simulink model "Timer_mdl"  (R2022b)
settings: Solver=FixedStepAuto  StartTime=0.0  StopTime=20  FixedStep=.01  RelTol=1e-3
settings Model: Creator=Sajjad  LastModifiedBy=Sajjad

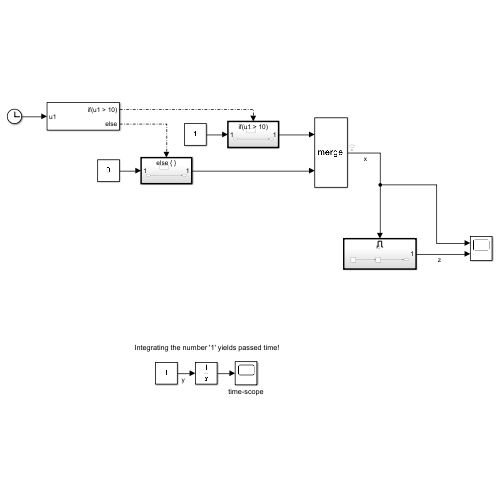
[thumbnail: Simulink's stored preview of the top-level diagram]
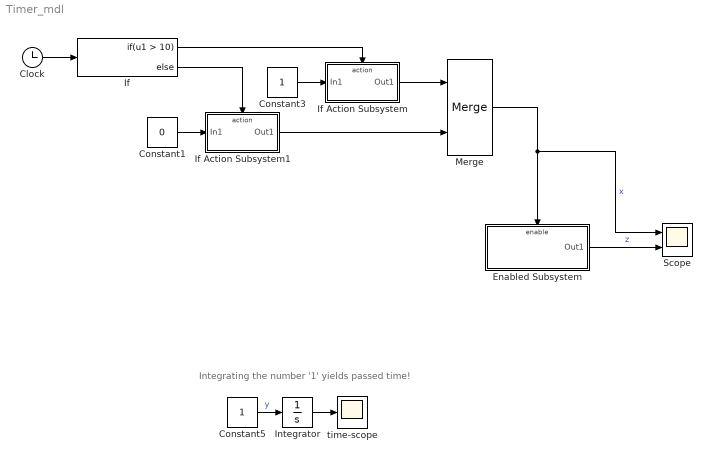
== system Timer_mdl ==
  note: Integrating the number '1' yields passed time!
  Clock : Clock
  Constant1 : Constant  Value=0
  Constant3 : Constant
  Constant5 : Constant
  Enabled Subsystem : Subsystem  TreatAsAtomicUnit=on
  If : If  IfExpression=u1 > 10
  If Action Subsystem : Subsystem  TreatAsAtomicUnit=on
  If Action Subsystem1 : Subsystem  TreatAsAtomicUnit=on
  Integrator : Integrator
  Merge : Merge
  Scope : Scope  NumInputPorts=2
  time-scope : Scope
  wires:
  Merge/1 -> Enabled Subsystem/Enable, Scope/1  "x"
  Clock/1 -> If/1
  If/1 -> If Action Subsystem/Action
  If/2 -> If Action Subsystem1/Action
  If Action Subsystem/1(Out1) -> Merge/1
  If Action Subsystem1/1(Out1) -> Merge/2
  Constant1/1 -> If Action Subsystem1/1(In1)
  Constant3/1 -> If Action Subsystem/1(In1)
  Constant5/1 -> Integrator/1  "y"
  Integrator/1 -> time-scope/1
  Enabled Subsystem/1(Out1) -> Scope/2  "z"

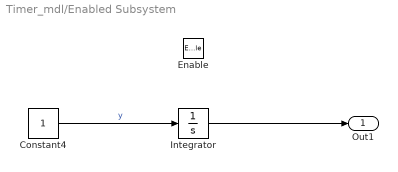
== system Timer_mdl/Enabled Subsystem ==
  Enable : EnablePort
  Constant4 : Constant
  Integrator : Integrator
  Out1 : Outport
  wires:
  Constant4/1 -> Integrator/1  "y"
  Integrator/1 -> Out1/1

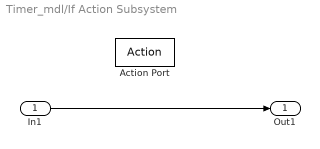
== system Timer_mdl/If Action Subsystem ==
  In1 : Inport
  Action Port : ActionPort  ActionPortLabel=if(u1 > 10)
  Out1 : Outport
  wires:
  In1/1 -> Out1/1

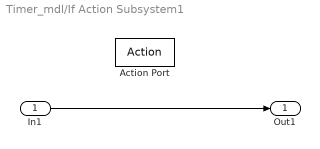
== system Timer_mdl/If Action Subsystem1 ==
  In1 : Inport
  Action Port : ActionPort  ActionPortLabel=else
  Out1 : Outport
  wires:
  In1/1 -> Out1/1
